simulink model "Final_Circuit"  (R2021b)
settings: Solver=VariableStepAuto  StartTime=0.0  StopTime=800  RelTol=1e-3
undefined symbols (not defined in the file): Ion, Lithium
libraries: spsSeriesRLCBranchLib x7, spsVoltageMeasurementLib x5, spsIdealSwitchLib x4, spsThyristorLib x4, spsCurrentMeasurementLib x3, spsACVoltageSourceLib x1, spsBatteryLib x1, spsDiodeLib x1, spsGroundLib x1, spsLinearTransformerLib x1, spsMosfetLib x1, spsSeriesRLCLoadLib x1
settings Model: Creator=Home  LastModifiedBy=SamZawad
settings SolverCC: AlgebraicLoopSolver=TrustRegion
settings DebuggingCC: SFMachineParentedDataDiag=warning

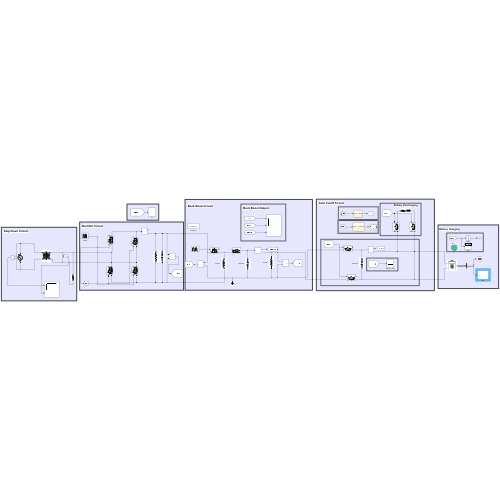
[thumbnail: Simulink's stored preview of the top-level diagram]
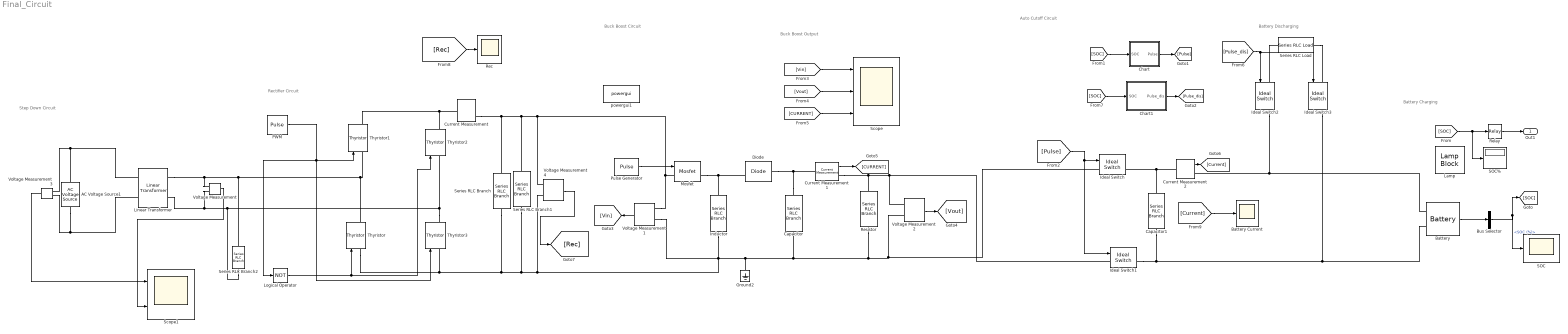
== system Final_Circuit ==
  note: Battery Charging
  note: Auto Cutoff Circuit
  note: Battery Discharging
  note: Buck Boost Circuit
  note: Buck Boost Output
  note: Rectifier Circuit
  note: Step Down Circuit
  AC Voltage Source1 : spsACVoltageSourceLib/AC Voltage Source  Amplitude=220  Phase=0  Frequency=50  SampleTime=0  Measurements=None  BusType=swing  Pref=10e3  Qref=0  Qmin=-inf  Qmax=+inf
  Battery : spsBatteryLib/Battery  BatType=Lithium-Ion  ShowTempParam=off  ThermalPreset=no  ShowAgeParam=off  NomV=7.2  NomQ=5.4  SOC=60  Batt_Tr=30  PresetModel=on  MaxQ=5.4  MinV=5.4  FullV=8.3807  Dis_rate=2.3478  R=0.013333  Normal_OP=4.8835  expZone="[7.7788      0.2653]"  current=[6.5 13 32.5]  Units=Time  Tci=20  NomT=20  T2=-30  MaxQ2=4.8  FullV2=7.1  Normal_OP2=5.655  expZone2="[6.58           1]"  Rca=0.6  ti=2000  Dp=0  Neq0=0  Tsim=1e6  Ta1=25  Qeol=5.4*0.9  Reol=0.013333*1.2  Char_age=[2.3478, 3]  Dis_age=[2.3478, 10]  N1=1500  N2=10500  N3=1000  N4=1400  Ta2=45  N5=950
  Battery Current : Scope
  Bus Selector : BusSelector  OutputSignals=SOC (%)
  Capacitor : spsSeriesRLCBranchLib/Series RLC Branch  LConnTagsString=__new0  RConnTagsString=__new0  BranchType=C  Resistance=1  Inductance=1e-3  SetiL0=off  InitialCurrent=0  Capacitance=0.08  Setx0=off  InitialVoltage=0  Measurements=None
  Capacitor1 : spsSeriesRLCBranchLib/Series RLC Branch  LConnTagsString=__new0  RConnTagsString=__new0  BranchType=C  Resistance=1  Inductance=1e-3  SetiL0=off  InitialCurrent=0  Capacitance=0.1  Setx0=off  InitialVoltage=0  Measurements=None
  Chart : Stateflow chart  TreatAsAtomicUnit=on
  Chart1 : Stateflow chart  TreatAsAtomicUnit=on
  Current Measurement : spsCurrentMeasurementLib/Current Measurement  PhasorSimulation=off  OutputType=Complex  PSBequivalent=0
  Current Measurement1 : spsCurrentMeasurementLib/Current Measurement  PhasorSimulation=off  OutputType=Complex  PSBequivalent=0
  Current Measurement2 : spsCurrentMeasurementLib/Current Measurement  PhasorSimulation=off  OutputType=Complex  PSBequivalent=0
  Diode : spsDiodeLib/Diode  Ron=0.001  Lon=0  Vf=0.8  IC=0  UseSnubber=0  Rs=500  Cs=250e-9  Measurements=on
  Ground2 : spsGroundLib/Ground  LConnTagsString=a
  Ideal Switch{,1..3} (4 alike) : spsIdealSwitchLib/Ideal Switch  Ron=0.001  Lon=0  IC=0  Rs=1e5  Cs=inf  Measurements=on
  Inductor : spsSeriesRLCBranchLib/Series RLC Branch  LConnTagsString=__new0  RConnTagsString=__new0  BranchType=L  Resistance=1  Inductance=100e-3  SetiL0=off  InitialCurrent=0  Capacitance=1e-6  Setx0=off  InitialVoltage=0  Measurements=None
  Lamp : LampBlock
  Linear Transformer : spsLinearTransformerLib/Linear Transformer  UNITS=pu  NominalPower=[ 250e6 60 ]  winding1="[ 220e3  0.002  0.08 ]"  winding2="[ 20e3  0.002  0.08 ]"  ThreeWindings=off  winding3=[ 315e3 0.002 0.08 ]  RmLm=[ 500 500 ]  Measurements=None  DataType=off
  Logical Operator : Logic  Operator=NOT  AllPortsSameDT=off  OutDataTypeStr=boolean
  Mosfet : spsMosfetLib/Mosfet  Ron=0.1  Lon=0  Rd=0.01  Vfd=0  IC=0  Rs=1e5  Cs=inf  Measurements=on
  PWM : DiscretePulseGenerator  PulseType=Time based  Period=0.02  PulseWidth=50
  Pulse Generator : DiscretePulseGenerator  PulseType=Time based  Period=1/100  PulseWidth=50
  Rec : Scope
  Relay : Relay  OnSwitchValue=80  OffSwitchValue=79
  Resistor : spsSeriesRLCBranchLib/Series RLC Branch  LConnTagsString=__new0  RConnTagsString=__new0  BranchType=R  Resistance=10  Inductance=1e-3  SetiL0=off  InitialCurrent=0  Capacitance=1e-6  Setx0=off  InitialVoltage=0  Measurements=None
  SOC : Scope
  SOC% : Display
  Scope : Scope  NumInputPorts=3
  Scope1 : Scope  NumInputPorts=2
  Series RLC Branch : spsSeriesRLCBranchLib/Series RLC Branch  LConnTagsString=__new0  RConnTagsString=__new0  BranchType=R  Resistance=100  Inductance=1e-3  SetiL0=off  InitialCurrent=0  Capacitance=1e-6  Setx0=off  InitialVoltage=0  Measurements=None
  Series RLC Branch1 : spsSeriesRLCBranchLib/Series RLC Branch  LConnTagsString=__new0  RConnTagsString=__new0  BranchType=C  Resistance=1  Inductance=1e-3  SetiL0=off  InitialCurrent=0  Capacitance=1  Setx0=off  InitialVoltage=0  Measurements=None
  Series RLC Branch2 : spsSeriesRLCBranchLib/Series RLC Branch  LConnTagsString=__new0  RConnTagsString=__new0  BranchType=R  Resistance=100  Inductance=1e-3  SetiL0=off  InitialCurrent=0  Capacitance=1e-6  Setx0=off  InitialVoltage=0  Measurements=None
  Series RLC Load : spsSeriesRLCLoadLib/Series RLC Load  LConnTagsString=a  RConnTagsString=__new0  NominalVoltage=10  NominalFrequency=60  ActivePower=1000  InductivePower=200  CapacitivePower=0  Setx0=off  InitialVoltage=0  SetiL0=off  InitialCurrent=0  Measurements=None  LoadType=constant Z
  Thyristor{,1..3} (4 alike) : spsThyristorLib/Thyristor  Ron=0.001  Lon=0  Vf=0.8  IC=0  Rs=500  Cs=250e-9  Measurements=on
  Voltage Measurement{,1..4} (5 alike) : spsVoltageMeasurementLib/Voltage Measurement  PhasorSimulation=off  OutputType=Complex  PSBequivalent=0
  powergui1 : spspowerguiLib/powergui  Priority=1  SimulationMode=Continuous  SampleTime=50e-6  frequency=60  Iterations=50  frequencyindice=50  Pbase=100e6  ErrMax=1e-4  UnitsV=kV  UnitsW=MW  buscounter=0  FunctionMessages=off  echomessages=off  EnableUseOfTLC=off  CurrentSourceSwitches=off  DisableSnubberDevices=off  DisableRonSwitches=off  DisableVfSwitches=off  DisplayEquations=off  AutomaticDiscreteSolvers=off  SolverType=Tustin/Backward Euler (TBE)  Interpol=off  ExternalGateDelay=off  methode=off  Ts=100  x0status=blocks  SPID=on  SwTol=0  HookPort=off  NonlinearTolerance=1e-4  nMaxIteration=100  ContinueOnMaxIteration=off  RestoreLinks=warning  ResistiveCurrentMeasurement=off  Frange=[0:2:500]  Ylog=off  Xlog=on  ShowGrid=off  save=off  variable=ZData  structure=0  ZoomFFT=off  StartTime=0.0  cycles=1  DisplayStyle=1  fundamental=60  FreqAxis=off  MaxFrequency=1000  frequencyindicesteady=1  RmsSteady=1  display=off
  Out1 : Outport
  wires:
  [SOC] -> Relay/1, SOC%/1
  Voltage Measurement1/1 -> [Vin]
  Battery/1 -> Bus Selector/1
  [SOC] -> Chart/1(SOC)
  [Vin] -> Scope/1
  Relay/1 -> Out1/1
  Pulse Generator/1 -> Mosfet/1
  [Pulse] -> Ideal Switch/1, Ideal Switch1/1
  [CURRENT] -> Scope/3
  Current Measurement1/1 -> [CURRENT]
  Bus Selector/1 -> SOC/1, [SOC]  "<SOC (%)>"
  [Vout] -> Scope/2
  Chart/1(Pulse) -> [Pulse]
  [Pulse_dis] -> Ideal Switch3/1, Ideal Switch2/1
  Chart1/1(Pulse_dis) -> [Pulse_dis]
  [SOC] -> Chart1/1(SOC)
  Voltage Measurement2/1 -> [Vout]
  [Current] -> Battery Current/1
  Current Measurement2/1 -> [Current]
  PWM/1 -> Logical Operator/1, Thyristor3/1, Thyristor1/1
  Logical Operator/1 -> Thyristor2/1, Thyristor/1
  Voltage Measurement3/1 -> Scope1/1
  Voltage Measurement/1 -> Scope1/2
  Voltage Measurement4/1 -> [Rec]
  [Rec] -> Rec/1
  connections:
  Capacitor/LConn1 -- Current Measurement1/LConn1 -- Diode/LConn1
  Inductor/LConn1 -- Diode/RConn1 -- Mosfet/RConn1
  Current Measurement1/RConn1 -- Ideal Switch1/LConn1 -- Voltage Measurement2/LConn1 -- Resistor/LConn1
  Current Measurement2/LConn1 -- Capacitor1/LConn1 -- Ideal Switch/RConn1
  Ideal Switch1/RConn1 -- Ideal Switch3/RConn1 -- Battery/LConn2 -- Capacitor1/RConn1
  Battery/LConn1 -- Ideal Switch2/RConn1 -- Current Measurement2/RConn1
  Series RLC Load/LConn1 -- Ideal Switch2/LConn1
  Series RLC Load/RConn1 -- Ideal Switch3/LConn1
  Thyristor/RConn1 -- Voltage Measurement/LConn1 -- Linear Transformer/RConn1 -- Series RLC Branch2/LConn1 -- Thyristor1/LConn1
  Thyristor1/RConn1 -- Current Measurement/LConn1 -- Thyristor2/RConn1
  Thyristor3/RConn1 -- Voltage Measurement/LConn2 -- Linear Transformer/RConn2 -- Series RLC Branch2/RConn1 -- Thyristor2/LConn1
  Current Measurement/RConn1 -- Voltage Measurement4/LConn1 -- Voltage Measurement1/LConn1 -- Mosfet/LConn1 -- Series RLC Branch1/LConn1 -- Series RLC Branch/LConn1
  Thyristor/LConn1 -- Ground2/LConn1 -- Ideal Switch/LConn1 -- Voltage Measurement2/LConn2 -- Resistor/RConn1 -- Capacitor/RConn1 -- Inductor/RConn1 -- Voltage Measurement1/LConn2 -- Voltage Measurement4/LConn2 -- Series RLC Branch1/RConn1 -- Series RLC Branch/RConn1 -- Thyristor3/LConn1
  AC Voltage Source1/RConn1 -- Voltage Measurement3/LConn2 -- Linear Transformer/LConn1
  AC Voltage Source1/LConn1 -- Voltage Measurement3/LConn1 -- Linear Transformer/LConn2

== stateflow chart Final_Circuit/Chart ==
  state Charge
    entry: Pulse=1
  state Discharge
    entry: Pulse=0
  (default) -> Charge
  Charge -> Discharge : [SOC>80]
  Discharge -> Charge : [SOC<40]
  data: SOC input; Pulse output

== stateflow chart Final_Circuit/Chart1 ==
  state Charge
    entry: Pulse_dis=0
  state Discharge
    entry: Pulse_dis=1
  (default) -> Charge
  Charge -> Discharge : [SOC>80]
  Discharge -> Charge : [SOC<40]
  data: SOC input; Pulse_dis output
